simulink model "buoy_FAM_sim_v2"  (R2023b)
settings: Solver=VariableStepAuto  StartTime=0.0  StopTime=60  MaxStep=0.01  RelTol=1e-3
model workspace (MAT data in the model file):
  CD_cmmt = Simulink.Parameter
  CD_cmmt.Value = 0.5
  CD_cmmt.DataType = 'auto'
  CD_cmmt.Complexity = 'real'
  CD_cmmt.Dimensions = [1 1]
  buoy_density_cmmt = Simulink.Parameter
  buoy_density_cmmt.Value = 881
  buoy_density_cmmt.Description = 'Set to match RM3 float weight of 207.6 Mg'
  buoy_density_cmmt.DataType = 'auto'
  buoy_density_cmmt.DocUnits = 'kg/m^3'
  buoy_density_cmmt.Complexity = 'real'
  buoy_density_cmmt.Dimensions = [1 1]
  buoy_height_cmmt = Simulink.Parameter
  buoy_height_cmmt.Value = 9
  buoy_height_cmmt.Description = 'Based on Sandia RM3 model'
  buoy_height_cmmt.DataType = 'auto'
  buoy_height_cmmt.DocUnits = 'm'
  buoy_height_cmmt.Complexity = 'real'
  buoy_height_cmmt.Dimensions = [1 1]
  buoy_radius_cmmt = Simulink.Parameter
  buoy_radius_cmmt.Value = 1.8
  buoy_radius_cmmt.Description = 'Based on Sandia RM3'
  buoy_radius_cmmt.DataType = 'auto'
  buoy_radius_cmmt.DocUnits = 'm'
  buoy_radius_cmmt.Complexity = 'real'
  buoy_radius_cmmt.Dimensions = [1 1]
  fluid_density = Simulink.Parameter
  fluid_density.Value = 1025
  fluid_density.DataType = 'auto'
  fluid_density.DocUnits = 'kg/m^3'
  fluid_density.Complexity = 'real'
  fluid_density.Dimensions = [1 1]
  gravity = Simulink.Parameter
  gravity.Value = 9.81
  gravity.DataType = 'auto'
  gravity.DocUnits = 'm/s^2'
  gravity.Complexity = 'real'
  gravity.Dimensions = [1 1]
  spring_const_cmmt = Simulink.Parameter
  spring_const_cmmt.Value = 1000
  spring_const_cmmt.DataType = 'auto'
  spring_const_cmmt.DocUnits = 'N/m'
  spring_const_cmmt.Complexity = 'real'
  spring_const_cmmt.Dimensions = [1 1]
  spring_unstretched_length = Simulink.Parameter
  spring_unstretched_length.Value = 0
  spring_unstretched_length.Description = 'Value of x where spring would have 0 force. Ex. with this set to -2, there would be 0 spring force if x=-2'
  spring_unstretched_length.DataType = 'auto'
  spring_unstretched_length.DocUnits = 'm'
  spring_unstretched_length.Complexity = 'real'
  spring_unstretched_length.Dimensions = [1 1]
  wave_amplitude_cmmt = Simulink.Parameter
  wave_amplitude_cmmt.Value = 1
  wave_amplitude_cmmt.DataType = 'auto'
  wave_amplitude_cmmt.DocUnits = 'm'
  wave_amplitude_cmmt.Complexity = 'real'
  wave_amplitude_cmmt.Dimensions = [1 1]
  wave_period_cmmt = Simulink.Parameter
  wave_period_cmmt.Value = 5
  wave_period_cmmt.DataType = 'auto'
  wave_period_cmmt.DocUnits = 's'
  wave_period_cmmt.Complexity = 'real'
  wave_period_cmmt.Dimensions = [1 1]
undefined symbols (not defined in the file): buoy_density, buoy_height, buoy_radius, CD, damping, spring_const, wave_amplitude, wave_period
libraries: FAM_lab_scale x1, FAM_simple_outflow x1, turbine_generator x1
settings Model: DataDictionary=FAM_parameters_lab_scale.sldd  Creator=Carson  LastModifiedBy=Carson
settings SimscapeCC: SimscapeLogType=all  SimscapeLogLimitData=off

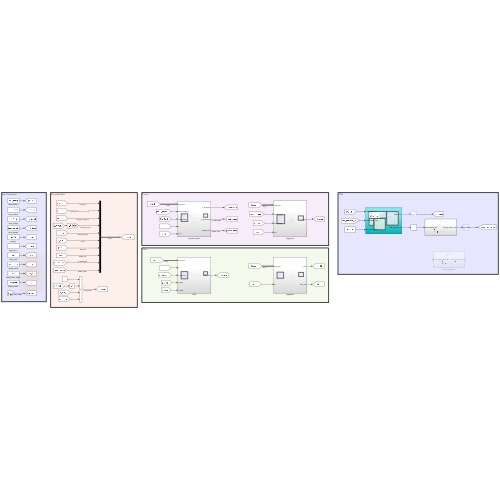
[thumbnail: Simulink's stored preview of the top-level diagram]
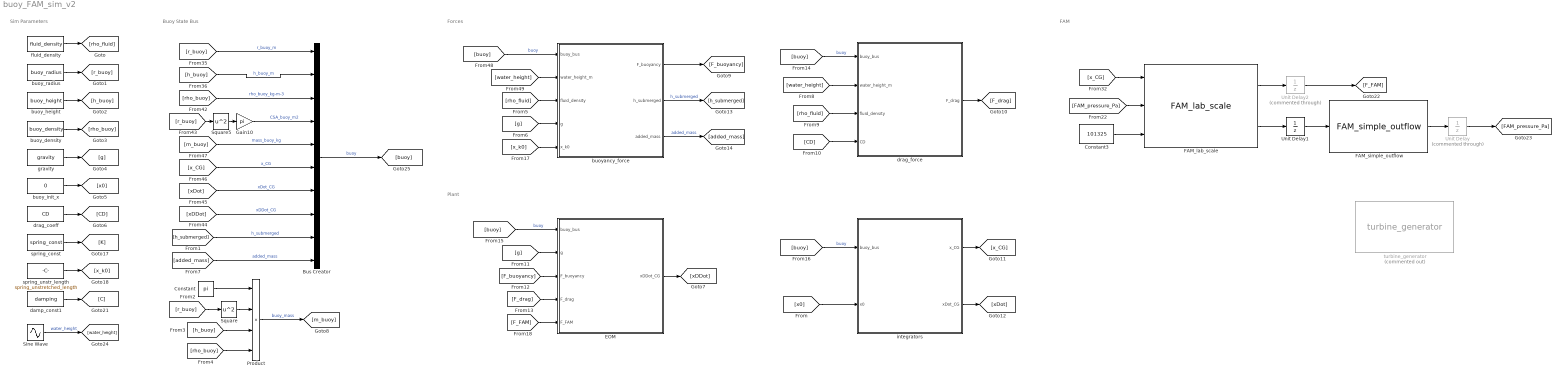
== system buoy_FAM_sim_v2 ==
  note: Plant
  note: Forces
  note: Buoy State Bus
  note: FAM
  note: Sim Parameters
  Bus Creator : BusCreator  Inputs=10
  Constant : Constant  Value=pi
  Constant3 : Constant  Value=101325
  EOM : Subsystem
  FAM_lab_scale : FAM_lab_scale/FAM_lab_scale  SystemSampleTime=-1  VariantActivationTime=update diagram  AllowFlexibleInterface=on  Latency=0  AutoFrameSizeCalculation=off
  FAM_simple_outflow : FAM_simple_outflow/FAM_simple_outflow  SystemSampleTime=-1  VariantActivationTime=update diagram  AllowFlexibleInterface=on  Latency=0  AutoFrameSizeCalculation=off
  Gain10 : Gain  Gain=pi
  Product : Product  Inputs=****
  Sine Wave : Sin  Amplitude=wave_amplitude  Frequency=2*pi/wave_period  SampleTime=0
  Square : Math  Operator=square
  Square5 : Math  Operator=square
  Unit Delay : UnitDelay  Commented=through  InitialCondition=101325  SampleTime=-1  HasFrameUpgradeWarning=on
  Unit Delay1 : UnitDelay  SampleTime=-1  HasFrameUpgradeWarning=on
  Unit Delay2 : UnitDelay  Commented=through  SampleTime=-1  HasFrameUpgradeWarning=on
  buoy_density : Constant  Value=buoy_density
  buoy_height : Constant  Value=buoy_height
  buoy_init_x : Constant  Value=0
  buoy_radius : Constant  Value=buoy_radius
  buoyancy_force : Subsystem
  damp_const1 : Constant  Value=damping
  drag_coeff : Constant  Value=CD
  drag_force : Subsystem
  fluid_density : Constant  Value=fluid_density
  gravity : Constant  Value=gravity
  integrators : Subsystem
  spring_const : Constant  Value=spring_const
  spring_unstr_length : Constant  Value=spring_unstretched_length
  turbine_generator : turbine_generator/turbine_generator  Commented=on  SystemSampleTime=-1  VariantActivationTime=update diagram  AllowFlexibleInterface=on  Latency=0  AutoFrameSizeCalculation=off
  wires:
  fluid_density/1 -> [rho_fluid]
  buoy_radius/1 -> [r_buoy]
  buoy_height/1 -> [h_buoy]
  buoy_density/1 -> [rho_buoy]
  gravity/1 -> [g]
  buoy_init_x/1 -> [x0]
  drag_coeff/1 -> [CD]
  spring_const/1 -> [K]
  spring_unstr_length/1 -> [x_k0]
  damp_const1/1 -> [C]
  FAM_lab_scale/1 -> Unit Delay2/1
  FAM_lab_scale/2 -> Unit Delay1/1
  FAM_simple_outflow/1 -> Unit Delay/1
  [FAM_pressure_Pa] -> FAM_lab_scale/2
  Constant3/1 -> FAM_lab_scale/3
  Unit Delay2/1 -> [F_FAM]
  [x_CG] -> FAM_lab_scale/1
  Sine Wave/1 -> [water_height]  "water_height"
  [x_CG] -> Bus Creator/6  "x_CG"
  Square5/1 -> Gain10/1
  [rho_buoy] -> Bus Creator/3  "rho_buoy_kg-m-3"
  Bus Creator/1 -> [buoy]  "buoy"
  [h_buoy] -> Bus Creator/2  "h_buoy_m"
  [xDot] -> Bus Creator/7  "xDot_CG"
  [r_buoy] -> Bus Creator/1  "r_buoy_m"
  [xDDot] -> Bus Creator/8  "xDDot_CG"
  [r_buoy] -> Square5/1
  Gain10/1 -> Bus Creator/4  "CSA_buoy_m2"
  Constant/1 -> Product/1
  [rho_buoy] -> Product/4
  Square/1 -> Product/2
  Product/1 -> [m_buoy]  "buoy_mass"
  [h_buoy] -> Product/3
  [r_buoy] -> Square/1
  [m_buoy] -> Bus Creator/5  "mass_buoy_kg"
  [buoy] -> buoyancy_force/1(buoy_bus)  "buoy"
  [water_height] -> buoyancy_force/2(water_height_m)
  [h_submerged] -> Bus Creator/9  "h_submerged"
  [rho_fluid] -> buoyancy_force/3(fluid_density)
  [added_mass] -> Bus Creator/10  "added_mass"
  [g] -> buoyancy_force/4(g)
  buoyancy_force/1(F_buoyancy) -> [F_buoyancy]
  [water_height] -> drag_force/2(water_height_m)
  [rho_fluid] -> drag_force/3(fluid_density)
  [CD] -> drag_force/4(CD)
  drag_force/1(F_drag) -> [F_drag]
  [g] -> EOM/2(g)
  [F_buoyancy] -> EOM/3(F_buoyancy)
  [F_drag] -> EOM/4(F_drag)
  [x0] -> integrators/2(x0)
  [F_FAM] -> EOM/5(F_FAM)
  integrators/1(x_CG) -> [x_CG]
  integrators/2(xDot_CG) -> [xDot]
  EOM/1(xDDot_CG) -> [xDDot]
  buoyancy_force/2(h_submerged) -> [h_submerged]  "h_submerged"
  buoyancy_force/3(added_mass) -> [added_mass]  "added_mass"
  [buoy] -> drag_force/1(buoy_bus)  "buoy"
  [buoy] -> EOM/1(buoy_bus)  "buoy"
  [buoy] -> integrators/1(buoy_bus)  "buoy"
  [x_k0] -> buoyancy_force/5(x_k0)
  Unit Delay/1 -> [FAM_pressure_Pa]
  Unit Delay1/1 -> FAM_simple_outflow/1

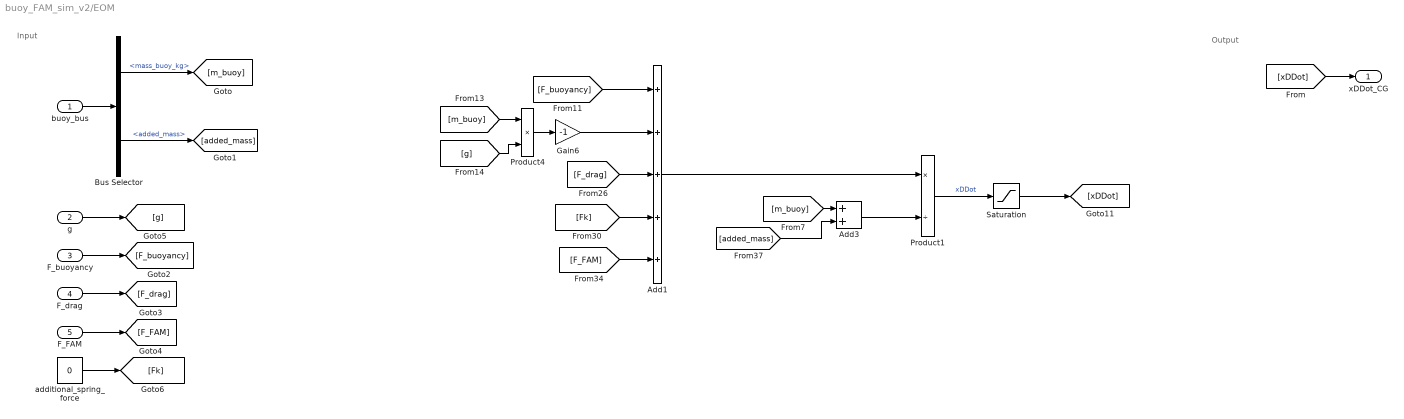
== system buoy_FAM_sim_v2/EOM ==
  note: Input
  note: Output
  buoy_bus : Inport
  g : Inport  Port=2
  F_buoyancy : Inport  Port=3
  F_drag : Inport  Port=4
  F_FAM : Inport  Port=5
  Add1 : Sum  Inputs=+++++
  Add3 : Sum
  Bus Selector : BusSelector  OutputSignals=mass_buoy_kg,added_mass
  Gain6 : Gain  Gain=-1
  Product1 : Product  Inputs=*/
  Product4 : Product
  Saturation : Saturate  UpperLimit=10  LowerLimit=-10
  additional_spring_force : Constant  Value=0
  xDDot_CG : Outport
  wires:
  Bus Selector/2 -> [added_mass]  "<added_mass>"
  Bus Selector/1 -> [m_buoy]  "<mass_buoy_kg>"
  buoy_bus/1 -> Bus Selector/1
  [F_buoyancy] -> Add1/1
  [m_buoy] -> Product4/1
  Add1/1 -> Product1/1
  [g] -> Product4/2
  [added_mass] -> Add3/2
  Product1/1 -> Saturation/1  "xDDot"
  [F_drag] -> Add1/3
  [F_FAM] -> Add1/5
  [m_buoy] -> Add3/1
  Add3/1 -> Product1/2
  Product4/1 -> Gain6/1
  [Fk] -> Add1/4
  Gain6/1 -> Add1/2
  g/1 -> [g]
  F_buoyancy/1 -> [F_buoyancy]
  F_drag/1 -> [F_drag]
  F_FAM/1 -> [F_FAM]
  additional_spring_force/1 -> [Fk]
  [xDDot] -> xDDot_CG/1
  Saturation/1 -> [xDDot]

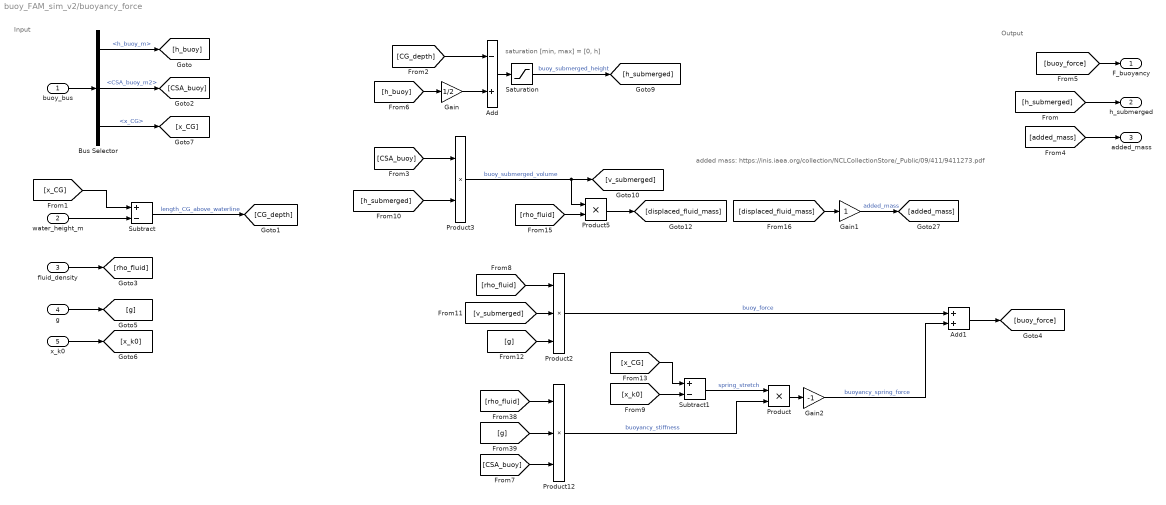
== system buoy_FAM_sim_v2/buoyancy_force ==
  note: Output
  note: Input
  note: saturation [min, max] = [0, h]
  note: added mass: https://inis.iaea.org/collection/NCLCollectionStore/_Public/09/411/9411273.pdf
  buoy_bus : Inport
  water_height_m : Inport  Port=2
  fluid_density : Inport  Port=3
  g : Inport  Port=4
  x_k0 : Inport  Port=5
  Add : Sum  Inputs=-+
  Add1 : Sum
  Bus Selector : BusSelector  OutputSignals=h_buoy_m,CSA_buoy_m2,x_CG
  Gain : Gain  Gain=1/2
  Gain1 : Gain
  Gain2 : Gain  Gain=-1
  Product : Product
  Product12 : Product  Inputs=***
  Product2 : Product  Inputs=***
  Product3 : Product  Inputs=**
  Product5 : Product
  Saturation : Saturate  UpperLimit=buoy_height  LowerLimit=0
  Subtract : Sum  Inputs=+-
  Subtract1 : Sum  Inputs=+-
  F_buoyancy : Outport
  h_submerged : Outport  Port=2
  added_mass : Outport  Port=3
  wires:
  Gain/1 -> Add/2
  [h_buoy] -> Gain/1
  Add/1 -> Saturation/1
  Saturation/1 -> [h_submerged]  "buoy_submerged_height"
  [CG_depth] -> Add/1
  [h_submerged] -> h_submerged/1
  [rho_fluid] -> Product5/2
  Product3/1 -> Product5/1, [v_submerged]  "buoy_submerged_volume"
  Product5/1 -> [displaced_fluid_mass]
  Gain1/1 -> [added_mass]  "added_mass"
  [displaced_fluid_mass] -> Gain1/1
  [h_submerged] -> Product3/2
  buoy_bus/1 -> Bus Selector/1
  Bus Selector/1 -> [h_buoy]  "<h_buoy_m>"
  Bus Selector/3 -> [x_CG]  "<x_CG>"
  water_height_m/1 -> Subtract/2
  [x_CG] -> Subtract/1
  Subtract/1 -> [CG_depth]  "length_CG_above_waterline"
  Bus Selector/2 -> [CSA_buoy]  "<CSA_buoy_m2>"
  [CSA_buoy] -> Product3/1
  fluid_density/1 -> [rho_fluid]
  [added_mass] -> added_mass/1
  [rho_fluid] -> Product2/1
  [g] -> Product2/3
  [v_submerged] -> Product2/2
  Product2/1 -> Add1/1  "buoy_force"
  [buoy_force] -> F_buoyancy/1
  g/1 -> [g]
  Product12/1 -> Product/2  "buoyancy_stiffness"
  [rho_fluid] -> Product12/1
  [g] -> Product12/2
  [CSA_buoy] -> Product12/3
  x_k0/1 -> [x_k0]
  [x_k0] -> Subtract1/2
  [x_CG] -> Subtract1/1
  Subtract1/1 -> Product/1  "spring_stretch"
  Product/1 -> Gain2/1
  Gain2/1 -> Add1/2  "buoyancy_spring_force"
  Add1/1 -> [buoy_force]

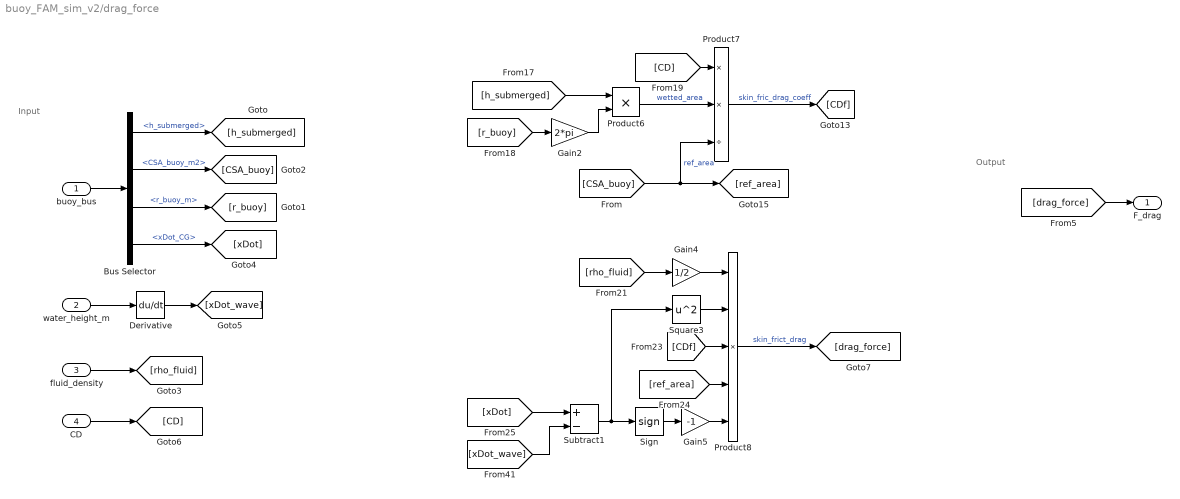
== system buoy_FAM_sim_v2/drag_force ==
  note: Input
  note: Output
  buoy_bus : Inport
  water_height_m : Inport  Port=2
  fluid_density : Inport  Port=3
  CD : Inport  Port=4
  Bus Selector : BusSelector  OutputSignals=h_submerged,CSA_buoy_m2,r_buoy_m,xDot_CG
  Derivative : Derivative
  Gain2 : Gain  Gain=2*pi
  Gain4 : Gain  Gain=1/2
  Gain5 : Gain  Gain=-1
  Product6 : Product
  Product7 : Product  Inputs=**/
  Product8 : Product  Inputs=*****
  Sign : Signum  ZeroCross=off
  Square3 : Math  Operator=square
  Subtract1 : Sum  Inputs=+-
  F_drag : Outport
  wires:
  [drag_force] -> F_drag/1
  Bus Selector/2 -> [CSA_buoy]  "<CSA_buoy_m2>"
  Bus Selector/4 -> [xDot]  "<xDot_CG>"
  Bus Selector/1 -> [h_submerged]  "<h_submerged>"
  buoy_bus/1 -> Bus Selector/1
  Gain2/1 -> Product6/2
  [h_submerged] -> Product6/1
  [CSA_buoy] -> [ref_area], Product7/3  "ref_area"
  [r_buoy] -> Gain2/1
  [CD] -> Product7/1
  Product6/1 -> Product7/2  "wetted_area"
  Product7/1 -> [CDf]  "skin_fric_drag_coeff"
  [xDot_wave] -> Subtract1/2
  [ref_area] -> Product8/4
  Square3/1 -> Product8/2
  Gain4/1 -> Product8/1
  Subtract1/1 -> Square3/1, Sign/1
  [xDot] -> Subtract1/1
  [CDf] -> Product8/3
  Gain5/1 -> Product8/5
  [rho_fluid] -> Gain4/1
  Sign/1 -> Gain5/1
  Product8/1 -> [drag_force]  "skin_frict_drag"
  Bus Selector/3 -> [r_buoy]  "<r_buoy_m>"
  fluid_density/1 -> [rho_fluid]
  water_height_m/1 -> Derivative/1
  Derivative/1 -> [xDot_wave]
  CD/1 -> [CD]

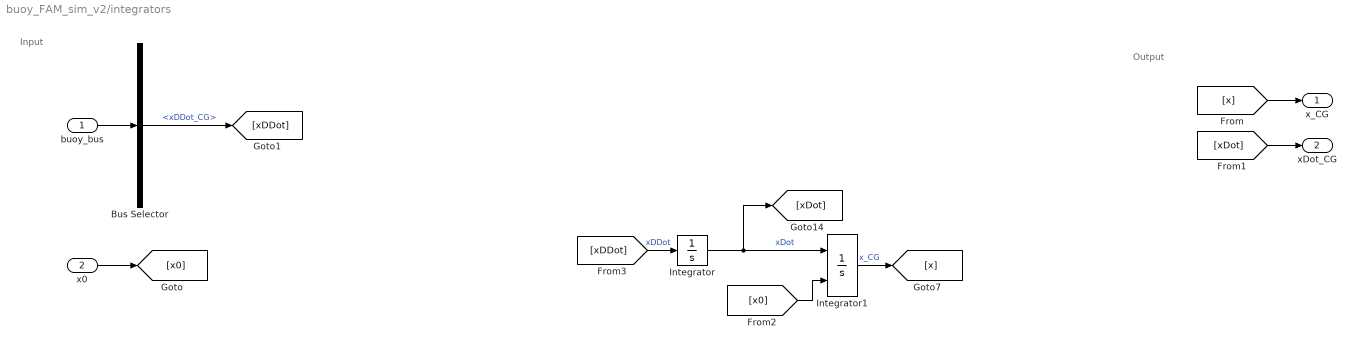
== system buoy_FAM_sim_v2/integrators ==
  note: Output
  note: Input
  buoy_bus : Inport
  x0 : Inport  Port=2
  Bus Selector : BusSelector  OutputSignals=xDDot_CG
  Integrator : Integrator
  Integrator1 : Integrator  InitialConditionSource=external
  x_CG : Outport
  xDot_CG : Outport  Port=2
  wires:
  [x] -> x_CG/1
  buoy_bus/1 -> Bus Selector/1
  [xDot] -> xDot_CG/1
  Integrator/1 -> [xDot], Integrator1/1  "xDot"
  Integrator1/1 -> [x]  "x_CG"
  [x0] -> Integrator1/2
  [xDDot] -> Integrator/1  "xDDot"
  x0/1 -> [x0]
  Bus Selector/1 -> [xDDot]  "<xDDot_CG>"
